simulink model "Query"  (R2013b)
settings: Solver=FixedStepDiscrete  StartTime=0.0  StopTime=30  FixedStep=Ts  RelTol=1e-3
InitFcn:
  | TeensyInit
StopFcn:
  | fopen(teensyConnection);
  | fwrite(teensyConnection,'S');
  | fclose(teensyConnection);
libraries: simulink x2, instrumentlib x1
settings Model: Creator=m2memari  LastModifiedBy=m2memari
settings DataIOCC: SignalLoggingSaveFormat=ModelDataLogs
settings DebuggingCC: MultiTaskDSMMsg=warning  MultiTaskCondExecSysMsg=none
settings RTWCC: IncludeERTFirstTime=on

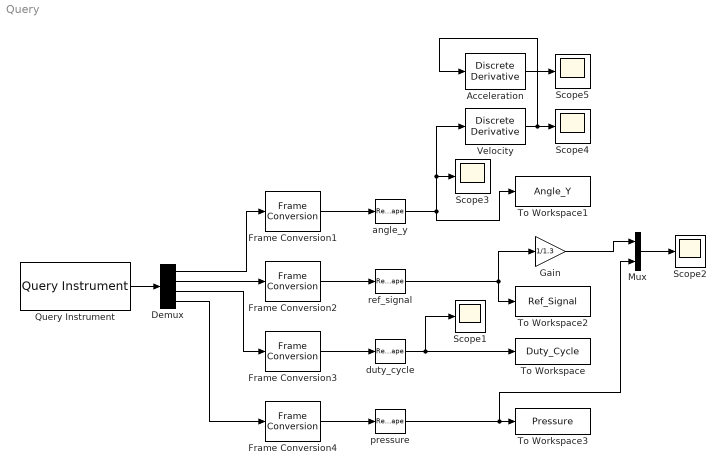
== system Query ==
  Acceleration : simulink/Discrete/Discrete Derivative  gainval=1.0  ICPrevScaledInput=0.0  InputProcessing=Inherited  OutMin=[]  OutMax=[]  OutDataType=fixdt(1, 16)  OutScaling=2^-10  DoSatur=off
  Demux : Demux
  Frame Conversion{1..4} (4 alike) : FrameConversion  OutFrame=Sample-based
  Gain : Gain  Gain=1/1.3
  Mux : Mux  Inputs=2
  Query Instrument : instrumentlib/Query Instrument  Priority=1  sampleTime=Ts  isWorkspaceObject=on  timeout=10  inputBufferSize=512  protocol=TCPIP  serialPort=COM1  baudRate=9600  gpibVendor=Advantech  boardIndex=0  primaryAddress=1  secondaryAddress=0  visaVendor=Agilent  visaSerialPort=0  chassisIndex=0  logicalAddress=0  tcpRemoteHost='127.0.0.1'  tcpRemotePort=28541  udpRemoteHost='127.0.0.1'  udpRemotePort=9090  visaTCPBoardIndex=0  visaTCPRemoteHost='127.0.0.1'  usbBoardIndex=0  usbManufID=0  usbModelCode=0  usbSerialNumber=0  wsVariableName=teensyConnection  initAction=Execute Function  initCommand='G'  initFunction=InitializeTeensy  queryCommand=''  responseFormat=ASCII  asciiFormatting='%g,%g,%g,%gy'  precision=8-bit integer  byteOrder=Little Endian  valuesToRead=1  removeBytes=off  afterOutputAction=Repeat query for new data  enableFrames=on  frameSize=4
  Scope{1..5} (5 alike) : Scope
      Scope1 settings: ShowLegends=on  TimeRange=10  YMin=0  YMax=2750
      Scope2 settings: ShowLegends=on  TimeRange=10  YMin=150  YMax=750  SaveName=ScopeData2
      Scope3 settings: ShowLegends=on  TimeRange=10  YMin=0  YMax=4.5  SaveName=ScopeData3
      Scope4 settings: ShowLegends=on  TimeRange=10  YMin=-40  YMax=40  SaveName=ScopeData4
      Scope5 settings: ShowLegends=on  TimeRange=10  YMin=-1000  YMax=1000  SaveName=ScopeData5
  To Workspace : ToWorkspace  VariableName=Duty_Cycle  SampleTime=-1  SaveFormat=Timeseries
  To Workspace1 : ToWorkspace  VariableName=Angle_Y  SampleTime=-1  SaveFormat=Timeseries
  To Workspace2 : ToWorkspace  VariableName=Ref_Signal  SampleTime=-1  SaveFormat=Timeseries
  To Workspace3 : ToWorkspace  VariableName=Pressure  SampleTime=-1  SaveFormat=Timeseries
  Velocity : simulink/Discrete/Discrete Derivative  gainval=1.0  ICPrevScaledInput=0.0  InputProcessing=Inherited  OutMin=[]  OutMax=[]  OutDataType=fixdt(1, 16)  OutScaling=2^-10  DoSatur=off
  angle_y : Reshape
  duty_cycle : Reshape
  pressure : Reshape
  ref_signal : Reshape
  wires:
  Frame Conversion1/1 -> angle_y/1
  Demux/1 -> Frame Conversion1/1
  Frame Conversion2/1 -> ref_signal/1
  Demux/2 -> Frame Conversion2/1
  Frame Conversion3/1 -> duty_cycle/1
  Demux/3 -> Frame Conversion3/1
  Frame Conversion4/1 -> pressure/1
  Demux/4 -> Frame Conversion4/1
  Query Instrument/1 -> Demux/1
  duty_cycle/1 -> To Workspace/1, Scope1/1
  angle_y/1 -> Velocity/1, Scope3/1, To Workspace1/1
  ref_signal/1 -> Gain/1, To Workspace2/1
  pressure/1 -> Mux/2, To Workspace3/1
  Velocity/1 -> Acceleration/1, Scope4/1
  Acceleration/1 -> Scope5/1
  Mux/1 -> Scope2/1
  Gain/1 -> Mux/1
